simulink model "PitchDynamics"  (R2014a)
settings: Solver=ode45  StartTime=0.0  StopTime=10.0  RelTol=1e-3
values from neighbouring files (symbols this model uses):
  a_theta1 = -rho*Va^2*c*S/(2*Jy)*Cm_q*c/(2*Va)    (= -14.426787663)    [MAINLongitudinal.m]
  a_theta2 = -rho*Va^2*c*S*Cm_alpha/(2*Jy)    (= 147.205731874)    [MAINLongitudinal.m]
  a_theta3 = rho*Va^2*c*S*Cm_deltaE/(2*Jy)    (= -165.053071401)    [MAINLongitudinal.m]
  kd_theta = (2*zeta_theta*w_ntheta-a_theta1)/a_theta3    [MAINLongitudinal.m]
  kp_theta = deltaElevator_max/e_thetamax*sign(a_theta3)    [MAINLongitudinal.m]
settings Model: Creator=Nathan  LastModifiedBy=Nathan

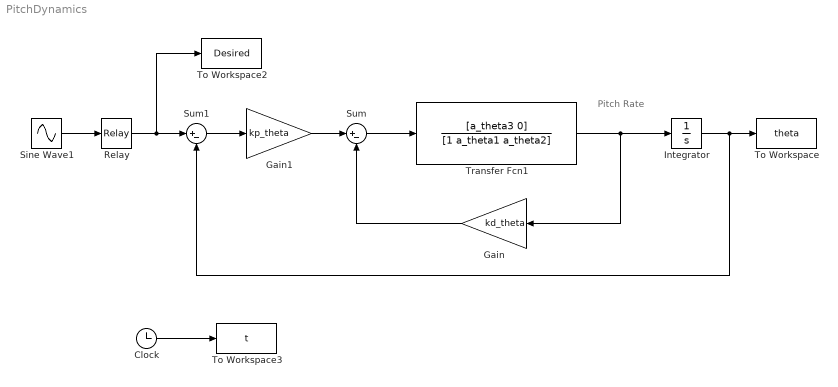
== system PitchDynamics ==
  note: Pitch Rate
  Clock : Clock
  Gain : Gain  Gain=kd_theta
  Gain1 : Gain  Gain=kp_theta
  Integrator : Integrator
  Relay : Relay  OffOutputValue=-1
  Sine Wave1 : Sin  SampleTime=0
  Sum : Sum  Inputs=|+-
  Sum1 : Sum  Inputs=|+-
  To Workspace : ToWorkspace  VariableName=theta  SampleTime=-1
  To Workspace2 : ToWorkspace  VariableName=Desired  SampleTime=-1
  To Workspace3 : ToWorkspace  VariableName=t  SampleTime=-1
  Transfer Fcn1 : TransferFcn  Numerator=[a_theta3 0]  Denominator=[1 a_theta1 a_theta2]
  wires:
  Transfer Fcn1/1 -> Integrator/1, Gain/1
  Gain/1 -> Sum/2
  Gain1/1 -> Sum/1
  Sum/1 -> Transfer Fcn1/1
  Integrator/1 -> To Workspace/1, Sum1/2
  Sum1/1 -> Gain1/1
  Sine Wave1/1 -> Relay/1
  Relay/1 -> To Workspace2/1, Sum1/1
  Clock/1 -> To Workspace3/1
